simulink model "template_81"  (R2024a)
settings: Solver=VariableStepAuto  StartTime=0.0  StopTime=10.0  RelTol=1e-3
model workspace (MATLAB code in the model file):
  | Kp = 2; % P-gain
  | Ti = 0.5; % Ti (integral time)
  | u_min = -1;
  | u_max = 1;
settings Model: Creator=chsl  LastModifiedBy=jacob
settings SolverCC: AlgebraicLoopSolver=TrustRegion
settings DebuggingCC: UnconnectedInputMsg=warning  UnconnectedOutputMsg=warning  UnconnectedLineMsg=warning
settings ModelReferenceCC: EnableRefExpFcnMdlSchedulingChecks=on
settings RTWCC: GPUComputeCapability=3.5  DLArmComputeVersion=19.05

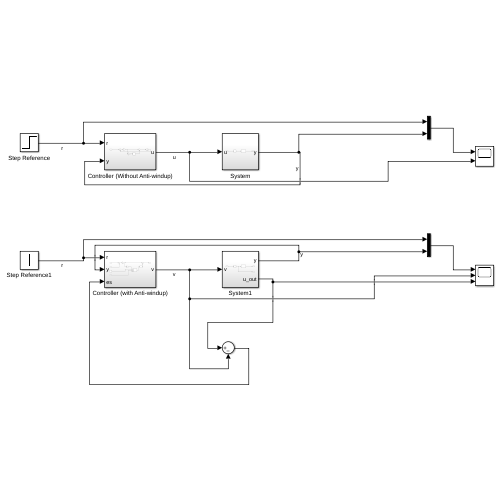
[thumbnail: Simulink's stored preview of the top-level diagram]
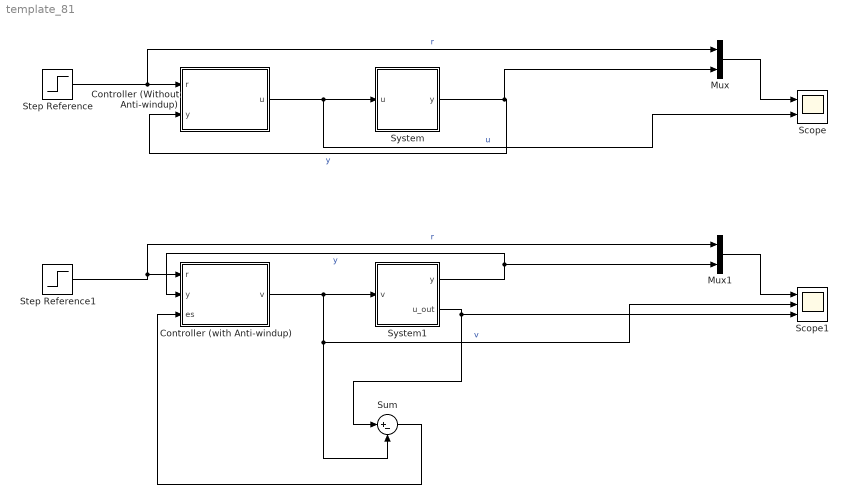
== system template_81 ==
  Controller (Without Anti-windup) : Subsystem
  Controller (with Anti-windup) : Subsystem
  Mux : Mux  Inputs=2
  Mux1 : Mux  Inputs=2
  Scope : Scope  NumInputPorts=2
  Scope1 : Scope  NumInputPorts=3
  Step Reference : Step  SampleTime=0
  Step Reference1 : Step  SampleTime=0
  Sum : Sum  Inputs=|+-
  System : Subsystem
  System1 : Subsystem
  wires:
  Step Reference/1 -> Mux/1, Controller (Without Anti-windup)/1(r)  "r"
  Controller (Without Anti-windup)/1(u) -> Scope/2, System/1(u)  "u"
  System/1(y) -> Mux/2, Controller (Without Anti-windup)/2(y)  "y"
  Mux/1 -> Scope/1
  System1/1(y) -> Controller (with Anti-windup)/2(y), Mux1/2  "y"
  Mux1/1 -> Scope1/1
  Controller (with Anti-windup)/1(v) -> Sum/2, Scope1/2, System1/1(v)  "v"
  Step Reference1/1 -> Mux1/1, Controller (with Anti-windup)/1(r)  "r"
  System1/2(u_out) -> Scope1/3, Sum/1
  Sum/1 -> Controller (with Anti-windup)/3(es)

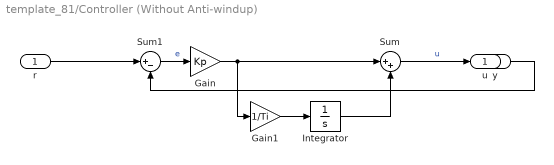
== system template_81/Controller (Without Anti-windup) ==
  r : Inport
  y : Inport  Port=2
  Gain : Gain  Gain=Kp
  Gain1 : Gain  Gain=1/Ti
  Integrator : Integrator
  Sum : Sum  Inputs=|++
  Sum1 : Sum  Inputs=|+-
  u : Outport
  wires:
  Sum/1 -> u/1  "u"
  Integrator/1 -> Sum/2
  Gain/1 -> Gain1/1, Sum/1
  y/1 -> Sum1/2
  Gain1/1 -> Integrator/1
  Sum1/1 -> Gain/1  "e"
  r/1 -> Sum1/1

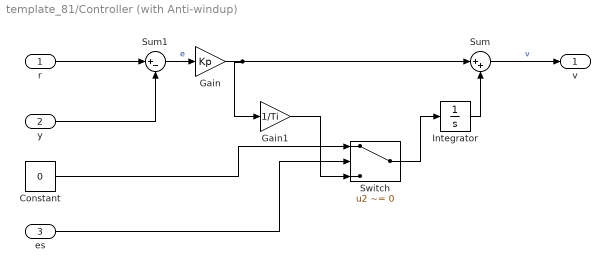
== system template_81/Controller (with Anti-windup) ==
  r : Inport
  y : Inport  Port=2
  es : Inport  Port=3
  Constant : Constant  Value=0
  Gain : Gain  Gain=Kp
  Gain1 : Gain  Gain=1/Ti
  Integrator : Integrator
  Sum : Sum  Inputs=|++
  Sum1 : Sum  Inputs=|+-
  Switch : Switch  Criteria=u2 ~= 0  SaturateOnIntegerOverflow=off  InputSameDT=off
  v : Outport
  wires:
  Sum/1 -> v/1  "v"
  Integrator/1 -> Sum/2
  Gain/1 -> Gain1/1, Sum/1
  y/1 -> Sum1/2
  Sum1/1 -> Gain/1  "e"
  r/1 -> Sum1/1
  es/1 -> Switch/2
  Switch/1 -> Integrator/1
  Constant/1 -> Switch/1
  Gain1/1 -> Switch/3

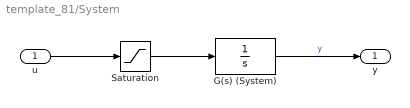
== system template_81/System ==
  u : Inport
  G(s) (System) : TransferFcn  Denominator=[1 0]
  Saturation : Saturate  UpperLimit=u_max  LowerLimit=u_min
  y : Outport
  wires:
  G(s) (System)/1 -> y/1  "y"
  u/1 -> Saturation/1
  Saturation/1 -> G(s) (System)/1

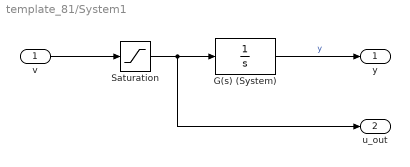
== system template_81/System1 ==
  v : Inport
  G(s) (System) : TransferFcn  Denominator=[1 0]
  Saturation : Saturate  UpperLimit=u_max  LowerLimit=u_min
  y : Outport
  u_out : Outport  Port=2
  wires:
  G(s) (System)/1 -> y/1  "y"
  v/1 -> Saturation/1
  Saturation/1 -> u_out/1, G(s) (System)/1
